simulink model "cps_4_11"  (R2016a)
settings: Solver=VariableStepAuto  StartTime=0.0  StopTime=10.0  RelTol=1e-3
undefined symbols (not defined in the file): sigbuilder_block
libraries: simulink x20
settings Model: Creator=benyett  LastModifiedBy=benyett

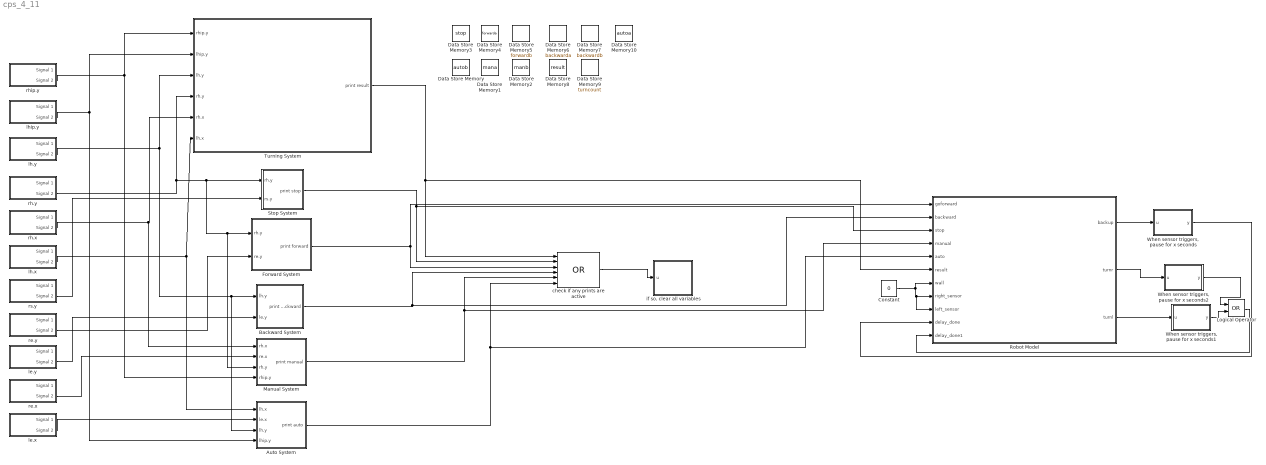
== system cps_4_11 ==
  Auto System : Subsystem
  Backward System : Subsystem
  Constant : Constant  Value=0
  Data Store Memory : DataStoreMemory  DataStoreName=autob  ReadBeforeWriteMsg=warning  WriteAfterWriteMsg=warning  WriteAfterReadMsg=warning  ShowAdditionalParam=off  OutDataTypeStr=double
  Data Store Memory1 : DataStoreMemory  DataStoreName=mana  ReadBeforeWriteMsg=warning  WriteAfterWriteMsg=warning  WriteAfterReadMsg=warning  ShowAdditionalParam=off  OutDataTypeStr=double
  Data Store Memory10 : DataStoreMemory  DataStoreName=autoa  ReadBeforeWriteMsg=warning  WriteAfterWriteMsg=warning  WriteAfterReadMsg=warning  ShowAdditionalParam=off  OutDataTypeStr=double
  Data Store Memory2 : DataStoreMemory  DataStoreName=manb  ReadBeforeWriteMsg=warning  WriteAfterWriteMsg=warning  WriteAfterReadMsg=warning  ShowAdditionalParam=off  OutDataTypeStr=double
  Data Store Memory3 : DataStoreMemory  DataStoreName=stop  ReadBeforeWriteMsg=warning  WriteAfterWriteMsg=warning  WriteAfterReadMsg=warning  ShowAdditionalParam=off  OutDataTypeStr=double
  Data Store Memory4 : DataStoreMemory  DataStoreName=forwarda  ReadBeforeWriteMsg=warning  WriteAfterWriteMsg=warning  WriteAfterReadMsg=warning  ShowAdditionalParam=off  OutDataTypeStr=double
  Data Store Memory5 : DataStoreMemory  DataStoreName=forwardb  ReadBeforeWriteMsg=warning  WriteAfterWriteMsg=warning  WriteAfterReadMsg=warning  ShowAdditionalParam=off  OutDataTypeStr=double
  Data Store Memory6 : DataStoreMemory  DataStoreName=backwarda  ReadBeforeWriteMsg=warning  WriteAfterWriteMsg=warning  WriteAfterReadMsg=warning  ShowAdditionalParam=off  OutDataTypeStr=double
  Data Store Memory7 : DataStoreMemory  DataStoreName=backwardb  ReadBeforeWriteMsg=warning  WriteAfterWriteMsg=warning  WriteAfterReadMsg=warning  ShowAdditionalParam=off  OutDataTypeStr=double
  Data Store Memory8 : DataStoreMemory  DataStoreName=result  ReadBeforeWriteMsg=warning  WriteAfterWriteMsg=warning  WriteAfterReadMsg=warning  ShowAdditionalParam=off  OutDataTypeStr=double
  Data Store Memory9 : DataStoreMemory  DataStoreName=turncount  ReadBeforeWriteMsg=warning  WriteAfterWriteMsg=warning  WriteAfterReadMsg=warning  ShowAdditionalParam=off  OutDataTypeStr=double
  Forward System : Subsystem
  Logical Operator : Logic  Operator=OR  AllPortsSameDT=off  OutDataTypeStr=boolean
  Manual System : Subsystem
  Robot Model : Stateflow chart  TreatAsAtomicUnit=on
  Stop System : Subsystem
  Turning System : Subsystem
  "When sensor triggers, pause for x seconds" : MATLAB Function  TreatAsAtomicUnit=on
  "When sensor triggers, pause for x seconds1" : MATLAB Function  TreatAsAtomicUnit=on
  "When sensor triggers, pause for x seconds2" : MATLAB Function  TreatAsAtomicUnit=on
  check if any prints are active : Logic  Operator=OR  Inputs=6  AllPortsSameDT=off  OutDataTypeStr=boolean
  "if so, clear all variables" : MATLAB Function  TreatAsAtomicUnit=on
  le.x : Subsystem  Tag=STV Subsys  LoadFcn=sigbuilder_block('load');  StartFcn=sigbuilder_block('start');  StopFcn=sigbuilder_block('stop');  ClipboardFcn=sigbuilder_block('clipboard');  mask(Sigbuilder block){}
      mask help: Simulink:masks:SigbuilderBlock_MD
      mask init:
      | if ~strcmp(get_param(bdroot(gcbh),'SimulationStatus'),'stopped') tuvar = sigbuilder_block('maskInit'); end
      settings: CopyFcn=sigbuilder_block('copy');  DeleteFcn=sigbuilder_block('delete');  ModelCloseFcn=sigbuilder_block('modelClose');  PreSaveFcn=sigbuilder_block('preSave');  PauseFcn=sigbuilder_block('pause');  ContinueFcn=sigbuilder_block('continue');  NameChangeFcn=sigbuilder_block('namechange');  OpenFcn=sigbuilder_block('open',[358 196 550 400 ]);  CloseFcn=sigbuilder_block('close');
      mask Display: plot(0, 0, 100, 100,[2, 2, 32, 32, 2], [68, 8, 8, 68, 68],[32, 2], [38, 38], [32, 19, 2],[53, 60, 44], [32, 17, 17, 2],[16, 16, 31, 31]);txt = getActiveGroup(gcbh);text(2, 100, txt,'verticalAlignment', 'top');
  le.y : Subsystem  Tag=STV Subsys  LoadFcn=sigbuilder_block('load');  StartFcn=sigbuilder_block('start');  StopFcn=sigbuilder_block('stop');  ClipboardFcn=sigbuilder_block('clipboard');  mask(Sigbuilder block){}
      mask help: Simulink:masks:SigbuilderBlock_MD
      mask init:
      | if ~strcmp(get_param(bdroot(gcbh),'SimulationStatus'),'stopped') tuvar = sigbuilder_block('maskInit'); end
      settings: CopyFcn=sigbuilder_block('copy');  DeleteFcn=sigbuilder_block('delete');  ModelCloseFcn=sigbuilder_block('modelClose');  PreSaveFcn=sigbuilder_block('preSave');  PauseFcn=sigbuilder_block('pause');  ContinueFcn=sigbuilder_block('continue');  NameChangeFcn=sigbuilder_block('namechange');  OpenFcn=sigbuilder_block('open',[358 196 550 400 ]);  CloseFcn=sigbuilder_block('close');
      mask Display: plot(0, 0, 100, 100,[2, 2, 32, 32, 2], [68, 8, 8, 68, 68],[32, 2], [38, 38], [32, 19, 2],[53, 60, 44], [32, 17, 17, 2],[16, 16, 31, 31]);txt = getActiveGroup(gcbh);text(2, 100, txt,'verticalAlignment', 'top');
  lh.x : Subsystem  Tag=STV Subsys  LoadFcn=sigbuilder_block('load');  StartFcn=sigbuilder_block('start');  StopFcn=sigbuilder_block('stop');  ClipboardFcn=sigbuilder_block('clipboard');  mask(Sigbuilder block){}
      mask help: Simulink:masks:SigbuilderBlock_MD
      mask init:
      | if ~strcmp(get_param(bdroot(gcbh),'SimulationStatus'),'stopped') tuvar = sigbuilder_block('maskInit'); end
      settings: CopyFcn=sigbuilder_block('copy');  DeleteFcn=sigbuilder_block('delete');  ModelCloseFcn=sigbuilder_block('modelClose');  PreSaveFcn=sigbuilder_block('preSave');  PauseFcn=sigbuilder_block('pause');  ContinueFcn=sigbuilder_block('continue');  NameChangeFcn=sigbuilder_block('namechange');  OpenFcn=sigbuilder_block('open',[358 196 550 400 ]);  CloseFcn=sigbuilder_block('close');
      mask Display: plot(0, 0, 100, 100,[2, 2, 32, 32, 2], [68, 8, 8, 68, 68],[32, 2], [38, 38], [32, 19, 2],[53, 60, 44], [32, 17, 17, 2],[16, 16, 31, 31]);txt = getActiveGroup(gcbh);text(2, 100, txt,'verticalAlignment', 'top');
  lh.y : Subsystem  Tag=STV Subsys  LoadFcn=sigbuilder_block('load');  StartFcn=sigbuilder_block('start');  StopFcn=sigbuilder_block('stop');  ClipboardFcn=sigbuilder_block('clipboard');  mask(Sigbuilder block){}
      mask help: Simulink:masks:SigbuilderBlock_MD
      mask init:
      | if ~strcmp(get_param(bdroot(gcbh),'SimulationStatus'),'stopped') tuvar = sigbuilder_block('maskInit'); end
      settings: CopyFcn=sigbuilder_block('copy');  DeleteFcn=sigbuilder_block('delete');  ModelCloseFcn=sigbuilder_block('modelClose');  PreSaveFcn=sigbuilder_block('preSave');  PauseFcn=sigbuilder_block('pause');  ContinueFcn=sigbuilder_block('continue');  NameChangeFcn=sigbuilder_block('namechange');  OpenFcn=sigbuilder_block('open',[358 196 550 400 ]);  CloseFcn=sigbuilder_block('close');
      mask Display: plot(0, 0, 100, 100,[2, 2, 32, 32, 2], [68, 8, 8, 68, 68],[32, 2], [38, 38], [32, 19, 2],[53, 60, 44], [32, 17, 17, 2],[16, 16, 31, 31]);txt = getActiveGroup(gcbh);text(2, 100, txt,'verticalAlignment', 'top');
  lhip.y : Subsystem  Tag=STV Subsys  LoadFcn=sigbuilder_block('load');  StartFcn=sigbuilder_block('start');  StopFcn=sigbuilder_block('stop');  ClipboardFcn=sigbuilder_block('clipboard');  mask(Sigbuilder block){}
      mask help: Simulink:masks:SigbuilderBlock_MD
      mask init:
      | if ~strcmp(get_param(bdroot(gcbh),'SimulationStatus'),'stopped') tuvar = sigbuilder_block('maskInit'); end
      settings: CopyFcn=sigbuilder_block('copy');  DeleteFcn=sigbuilder_block('delete');  ModelCloseFcn=sigbuilder_block('modelClose');  PreSaveFcn=sigbuilder_block('preSave');  PauseFcn=sigbuilder_block('pause');  ContinueFcn=sigbuilder_block('continue');  NameChangeFcn=sigbuilder_block('namechange');  OpenFcn=sigbuilder_block('open',[358 196 550 400 ]);  CloseFcn=sigbuilder_block('close');
      mask Display: plot(0, 0, 100, 100,[2, 2, 32, 32, 2], [68, 8, 8, 68, 68],[32, 2], [38, 38], [32, 19, 2],[53, 60, 44], [32, 17, 17, 2],[16, 16, 31, 31]);txt = getActiveGroup(gcbh);text(2, 100, txt,'verticalAlignment', 'top');
  re.x : Subsystem  Tag=STV Subsys  LoadFcn=sigbuilder_block('load');  StartFcn=sigbuilder_block('start');  StopFcn=sigbuilder_block('stop');  ClipboardFcn=sigbuilder_block('clipboard');  mask(Sigbuilder block){}
      mask help: Simulink:masks:SigbuilderBlock_MD
      mask init:
      | if ~strcmp(get_param(bdroot(gcbh),'SimulationStatus'),'stopped') tuvar = sigbuilder_block('maskInit'); end
      settings: CopyFcn=sigbuilder_block('copy');  DeleteFcn=sigbuilder_block('delete');  ModelCloseFcn=sigbuilder_block('modelClose');  PreSaveFcn=sigbuilder_block('preSave');  PauseFcn=sigbuilder_block('pause');  ContinueFcn=sigbuilder_block('continue');  NameChangeFcn=sigbuilder_block('namechange');  OpenFcn=sigbuilder_block('open',[358 196 550 400 ]);  CloseFcn=sigbuilder_block('close');
      mask Display: plot(0, 0, 100, 100,[2, 2, 32, 32, 2], [68, 8, 8, 68, 68],[32, 2], [38, 38], [32, 19, 2],[53, 60, 44], [32, 17, 17, 2],[16, 16, 31, 31]);txt = getActiveGroup(gcbh);text(2, 100, txt,'verticalAlignment', 'top');
  re.y : Subsystem  Tag=STV Subsys  LoadFcn=sigbuilder_block('load');  StartFcn=sigbuilder_block('start');  StopFcn=sigbuilder_block('stop');  ClipboardFcn=sigbuilder_block('clipboard');  mask(Sigbuilder block){}
      mask help: Simulink:masks:SigbuilderBlock_MD
      mask init:
      | if ~strcmp(get_param(bdroot(gcbh),'SimulationStatus'),'stopped') tuvar = sigbuilder_block('maskInit'); end
      settings: CopyFcn=sigbuilder_block('copy');  DeleteFcn=sigbuilder_block('delete');  ModelCloseFcn=sigbuilder_block('modelClose');  PreSaveFcn=sigbuilder_block('preSave');  PauseFcn=sigbuilder_block('pause');  ContinueFcn=sigbuilder_block('continue');  NameChangeFcn=sigbuilder_block('namechange');  OpenFcn=sigbuilder_block('open',[358 196 550 400 ]);  CloseFcn=sigbuilder_block('close');
      mask Display: plot(0, 0, 100, 100,[2, 2, 32, 32, 2], [68, 8, 8, 68, 68],[32, 2], [38, 38], [32, 19, 2],[53, 60, 44], [32, 17, 17, 2],[16, 16, 31, 31]);txt = getActiveGroup(gcbh);text(2, 100, txt,'verticalAlignment', 'top');
  rh.x : Subsystem  Tag=STV Subsys  LoadFcn=sigbuilder_block('load');  StartFcn=sigbuilder_block('start');  StopFcn=sigbuilder_block('stop');  ClipboardFcn=sigbuilder_block('clipboard');  mask(Sigbuilder block){}
      mask help: Simulink:masks:SigbuilderBlock_MD
      mask init:
      | if ~strcmp(get_param(bdroot(gcbh),'SimulationStatus'),'stopped') tuvar = sigbuilder_block('maskInit'); end
      settings: CopyFcn=sigbuilder_block('copy');  DeleteFcn=sigbuilder_block('delete');  ModelCloseFcn=sigbuilder_block('modelClose');  PreSaveFcn=sigbuilder_block('preSave');  PauseFcn=sigbuilder_block('pause');  ContinueFcn=sigbuilder_block('continue');  NameChangeFcn=sigbuilder_block('namechange');  OpenFcn=sigbuilder_block('open',[358 196 550 400 ]);  CloseFcn=sigbuilder_block('close');
      mask Display: plot(0, 0, 100, 100,[2, 2, 32, 32, 2], [68, 8, 8, 68, 68],[32, 2], [38, 38], [32, 19, 2],[53, 60, 44], [32, 17, 17, 2],[16, 16, 31, 31]);txt = getActiveGroup(gcbh);text(2, 100, txt,'verticalAlignment', 'top');
  rh.y : Subsystem  Tag=STV Subsys  LoadFcn=sigbuilder_block('load');  StartFcn=sigbuilder_block('start');  StopFcn=sigbuilder_block('stop');  ClipboardFcn=sigbuilder_block('clipboard');  mask(Sigbuilder block){}
      mask help: Simulink:masks:SigbuilderBlock_MD
      mask init:
      | if ~strcmp(get_param(bdroot(gcbh),'SimulationStatus'),'stopped') tuvar = sigbuilder_block('maskInit'); end
      settings: CopyFcn=sigbuilder_block('copy');  DeleteFcn=sigbuilder_block('delete');  ModelCloseFcn=sigbuilder_block('modelClose');  PreSaveFcn=sigbuilder_block('preSave');  PauseFcn=sigbuilder_block('pause');  ContinueFcn=sigbuilder_block('continue');  NameChangeFcn=sigbuilder_block('namechange');  OpenFcn=sigbuilder_block('open',[358 196 550 400 ]);  CloseFcn=sigbuilder_block('close');
      mask Display: plot(0, 0, 100, 100,[2, 2, 32, 32, 2], [68, 8, 8, 68, 68],[32, 2], [38, 38], [32, 19, 2],[53, 60, 44], [32, 17, 17, 2],[16, 16, 31, 31]);txt = getActiveGroup(gcbh);text(2, 100, txt,'verticalAlignment', 'top');
  rhip.y : Subsystem  Tag=STV Subsys  LoadFcn=sigbuilder_block('load');  StartFcn=sigbuilder_block('start');  StopFcn=sigbuilder_block('stop');  ClipboardFcn=sigbuilder_block('clipboard');  mask(Sigbuilder block){}
      mask help: Simulink:masks:SigbuilderBlock_MD
      mask init:
      | if ~strcmp(get_param(bdroot(gcbh),'SimulationStatus'),'stopped') tuvar = sigbuilder_block('maskInit'); end
      settings: CopyFcn=sigbuilder_block('copy');  DeleteFcn=sigbuilder_block('delete');  ModelCloseFcn=sigbuilder_block('modelClose');  PreSaveFcn=sigbuilder_block('preSave');  PauseFcn=sigbuilder_block('pause');  ContinueFcn=sigbuilder_block('continue');  NameChangeFcn=sigbuilder_block('namechange');  OpenFcn=sigbuilder_block('open',[358 196 550 400 ]);  CloseFcn=sigbuilder_block('close');
      mask Display: plot(0, 0, 100, 100,[2, 2, 32, 32, 2], [68, 8, 8, 68, 68],[32, 2], [38, 38], [32, 19, 2],[53, 60, 44], [32, 17, 17, 2],[16, 16, 31, 31]);txt = getActiveGroup(gcbh);text(2, 100, txt,'verticalAlignment', 'top');
  rs.y : Subsystem  Tag=STV Subsys  LoadFcn=sigbuilder_block('load');  StartFcn=sigbuilder_block('start');  StopFcn=sigbuilder_block('stop');  ClipboardFcn=sigbuilder_block('clipboard');  mask(Sigbuilder block){}
      mask help: Simulink:masks:SigbuilderBlock_MD
      mask init:
      | if ~strcmp(get_param(bdroot(gcbh),'SimulationStatus'),'stopped') tuvar = sigbuilder_block('maskInit'); end
      settings: CopyFcn=sigbuilder_block('copy');  DeleteFcn=sigbuilder_block('delete');  ModelCloseFcn=sigbuilder_block('modelClose');  PreSaveFcn=sigbuilder_block('preSave');  PauseFcn=sigbuilder_block('pause');  ContinueFcn=sigbuilder_block('continue');  NameChangeFcn=sigbuilder_block('namechange');  OpenFcn=sigbuilder_block('open',[358 196 550 400 ]);  CloseFcn=sigbuilder_block('close');
      mask Display: plot(0, 0, 100, 100,[2, 2, 32, 32, 2], [68, 8, 8, 68, 68],[32, 2], [38, 38], [32, 19, 2],[53, 60, 44], [32, 17, 17, 2],[16, 16, 31, 31]);txt = getActiveGroup(gcbh);text(2, 100, txt,'verticalAlignment', 'top');
  wires:
  Turning System/1(print result) -> Robot Model/6(result), check if any prints are active/1
  Stop System/1(print stop) -> Robot Model/3(stop), check if any prints are active/2
  Forward System/1(print forward) -> Robot Model/1(goforward), check if any prints are active/3
  Backward System/1(print backward) -> Robot Model/2(backward), check if any prints are active/4
  Manual System/1(print manual) -> Robot Model/4(manual), check if any prints are active/5
  Auto System/1(print auto) -> Robot Model/5(auto), check if any prints are active/6
  check if any prints are active/1 -> "if so, clear all variables"/1(u)
  rhip.y/2(Signal 2) -> Manual System/4(rhip.y), Turning System/1(rhip.y)
  lhip.y/2(Signal 2) -> Auto System/4(lhip.y), Turning System/2(lhip.y)
  lh.y/2(Signal 2) -> Auto System/3(lh.y), Backward System/1(lh.y), Turning System/3(lh.y)
  rh.y/2(Signal 2) -> Manual System/3(rh.y), Forward System/1(rh.y), Stop System/1(rh.y), Turning System/4(rh.y)
  rh.x/2(Signal 2) -> Manual System/1(rh.x), Turning System/5(rh.x)
  lh.x/2(Signal 2) -> Auto System/1(lh.x), Turning System/6(lh.x)
  rs.y/2(Signal 2) -> Stop System/2(rs.y)
  re.y/2(Signal 2) -> Forward System/2(re.y)
  le.y/2(Signal 2) -> Backward System/2(le.y)
  re.x/2(Signal 2) -> Manual System/2(re.x)
  le.x/2(Signal 2) -> Auto System/2(le.x)
  "When sensor triggers, pause for x seconds"/1(y) -> Robot Model/10(delay_done)
  Robot Model/1(backup) -> "When sensor triggers, pause for x seconds"/1(u)
  Robot Model/2(turnr) -> "When sensor triggers, pause for x seconds2"/1(u)
  Robot Model/3(turnl) -> "When sensor triggers, pause for x seconds1"/1(u)
  Constant/1 -> Robot Model/9(left_sensor), Robot Model/8(right_sensor), Robot Model/7(wall)
  "When sensor triggers, pause for x seconds2"/1(y) -> Logical Operator/1
  "When sensor triggers, pause for x seconds1"/1(y) -> Logical Operator/2
  Logical Operator/1 -> Robot Model/11(delay_done1)

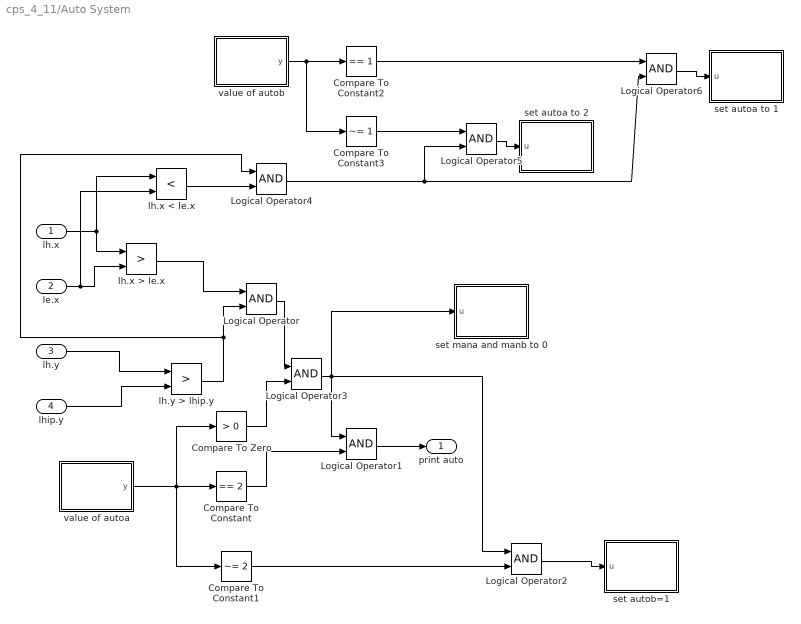
== system cps_4_11/Auto System ==
  lh.x : Inport
  le.x : Inport  Port=2
  lh.y : Inport  Port=3
  lhip.y : Inport  Port=4
  Compare To Constant : simulink/Logic and Bit Operations/Compare To Constant  relop===  const=2  OutDataTypeStr=boolean
  Compare To Constant1 : simulink/Logic and Bit Operations/Compare To Constant  relop=~=  const=2  OutDataTypeStr=boolean
  Compare To Constant2 : simulink/Logic and Bit Operations/Compare To Constant  relop===  const=1  OutDataTypeStr=boolean
  Compare To Constant3 : simulink/Logic and Bit Operations/Compare To Constant  relop=~=  const=1  OutDataTypeStr=boolean
  Compare To Zero : simulink/Logic and Bit Operations/Compare To Zero  relop=>  OutDataTypeStr=boolean
  Logical Operator{,1..6} (7 alike) : Logic  AllPortsSameDT=off  OutDataTypeStr=boolean
  lh.x < le.x : RelationalOperator  Operator=<  OutDataTypeStr=boolean
  lh.x > le.x : RelationalOperator  Operator=>  OutDataTypeStr=boolean
  lh.y > lhip.y : RelationalOperator  Operator=>  OutDataTypeStr=boolean
  set autoa to 1 : MATLAB Function  TreatAsAtomicUnit=on
  set autoa to 2 : MATLAB Function  TreatAsAtomicUnit=on
  set autob=1 : MATLAB Function  TreatAsAtomicUnit=on
  set mana and manb to 0 : MATLAB Function  TreatAsAtomicUnit=on
  value of autoa : MATLAB Function  TreatAsAtomicUnit=on
  value of autob : MATLAB Function  TreatAsAtomicUnit=on
  print auto : Outport
  wires:
  le.x/1 -> lh.x < le.x/2, lh.x > le.x/2
  lh.x/1 -> lh.x < le.x/1, lh.x > le.x/1
  lhip.y/1 -> lh.y > lhip.y/2
  lh.y/1 -> lh.y > lhip.y/1
  lh.x > le.x/1 -> Logical Operator/1
  lh.y > lhip.y/1 -> Logical Operator4/1, Logical Operator/2
  Logical Operator/1 -> Logical Operator3/1
  value of autoa/1(y) -> Compare To Zero/1, Compare To Constant1/1, Compare To Constant/1
  Compare To Constant/1 -> Logical Operator1/2
  Compare To Constant1/1 -> Logical Operator2/2
  Logical Operator1/1 -> print auto/1
  Logical Operator2/1 -> set autob=1/1(u)
  Logical Operator3/1 -> set mana and manb to 0/1(u), Logical Operator1/1, Logical Operator2/1
  Compare To Zero/1 -> Logical Operator3/2
  lh.x < le.x/1 -> Logical Operator4/2
  value of autob/1(y) -> Compare To Constant3/1, Compare To Constant2/1
  Compare To Constant3/1 -> Logical Operator5/1
  Compare To Constant2/1 -> Logical Operator6/1
  Logical Operator4/1 -> Logical Operator5/2, Logical Operator6/2
  Logical Operator5/1 -> set autoa to 2/1(u)
  Logical Operator6/1 -> set autoa to 1/1(u)

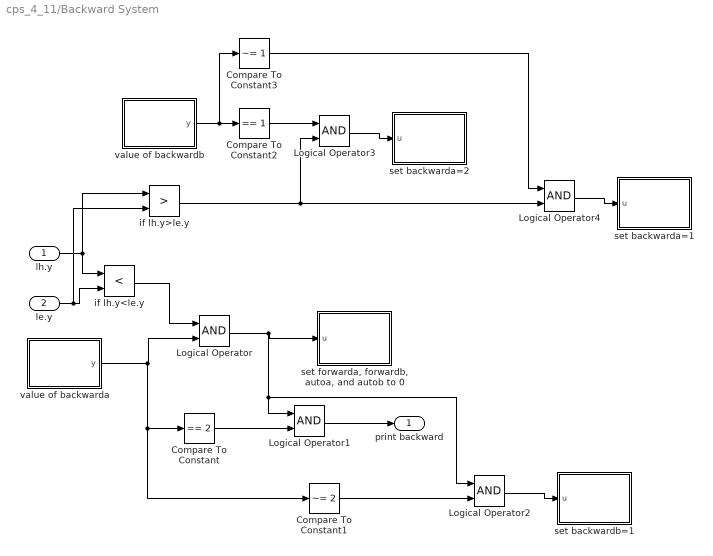
== system cps_4_11/Backward System ==
  lh.y : Inport
  le.y : Inport  Port=2
  Compare To Constant : simulink/Logic and Bit Operations/Compare To Constant  relop===  const=2  OutDataTypeStr=boolean
  Compare To Constant1 : simulink/Logic and Bit Operations/Compare To Constant  relop=~=  const=2  OutDataTypeStr=boolean
  Compare To Constant2 : simulink/Logic and Bit Operations/Compare To Constant  relop===  const=1  OutDataTypeStr=boolean
  Compare To Constant3 : simulink/Logic and Bit Operations/Compare To Constant  relop=~=  const=1  OutDataTypeStr=boolean
  Logical Operator{,1..4} (5 alike) : Logic  AllPortsSameDT=off  OutDataTypeStr=boolean
  if lh.y<le.y : RelationalOperator  Operator=<  OutDataTypeStr=boolean
  if lh.y>le.y : RelationalOperator  Operator=>  OutDataTypeStr=boolean
  set backwarda=1 : MATLAB Function  TreatAsAtomicUnit=on
  set backwarda=2 : MATLAB Function  TreatAsAtomicUnit=on
  set backwardb=1 : MATLAB Function  TreatAsAtomicUnit=on
  "set forwarda, forwardb, autoa, and autob to 0" : MATLAB Function  TreatAsAtomicUnit=on
  value of backwarda : MATLAB Function  TreatAsAtomicUnit=on
  value of backwardb : MATLAB Function  TreatAsAtomicUnit=on
  print backward : Outport
  wires:
  le.y/1 -> if lh.y>le.y/2, if lh.y<le.y/2
  lh.y/1 -> if lh.y>le.y/1, if lh.y<le.y/1
  if lh.y<le.y/1 -> Logical Operator/1
  value of backwarda/1(y) -> Compare To Constant1/1, Compare To Constant/1, Logical Operator/2
  Logical Operator/1 -> Logical Operator2/1, Logical Operator1/1, "set forwarda, forwardb, autoa, and autob to 0"/1(u)
  Compare To Constant/1 -> Logical Operator1/2
  Logical Operator1/1 -> print backward/1
  Compare To Constant1/1 -> Logical Operator2/2
  Logical Operator2/1 -> set backwardb=1/1(u)
  value of backwardb/1(y) -> Compare To Constant3/1, Compare To Constant2/1
  if lh.y>le.y/1 -> Logical Operator3/2, Logical Operator4/2
  Compare To Constant2/1 -> Logical Operator3/1
  Compare To Constant3/1 -> Logical Operator4/1
  Logical Operator4/1 -> set backwarda=1/1(u)
  Logical Operator3/1 -> set backwarda=2/1(u)

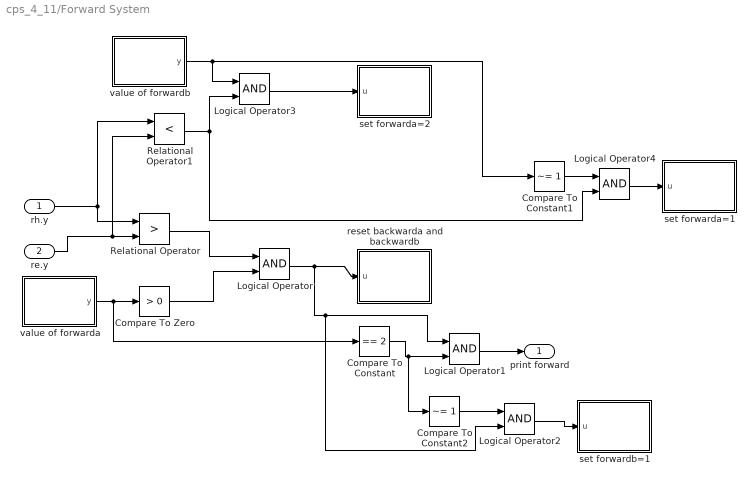
== system cps_4_11/Forward System ==
  rh.y : Inport
  re.y : Inport  Port=2
  Compare To Constant : simulink/Logic and Bit Operations/Compare To Constant  relop===  const=2  OutDataTypeStr=boolean
  Compare To Constant1 : simulink/Logic and Bit Operations/Compare To Constant  relop=~=  const=1  OutDataTypeStr=boolean
  Compare To Constant2 : simulink/Logic and Bit Operations/Compare To Constant  relop=~=  const=1  OutDataTypeStr=boolean
  Compare To Zero : simulink/Logic and Bit Operations/Compare To Zero  relop=>  OutDataTypeStr=boolean
  Logical Operator{,1..4} (5 alike) : Logic  AllPortsSameDT=off  OutDataTypeStr=boolean
  Relational Operator : RelationalOperator  Operator=>  OutDataTypeStr=boolean
  Relational Operator1 : RelationalOperator  Operator=<  OutDataTypeStr=boolean
  reset backwarda and backwardb : MATLAB Function  TreatAsAtomicUnit=on
  set forwarda=1 : MATLAB Function  TreatAsAtomicUnit=on
  set forwarda=2 : MATLAB Function  TreatAsAtomicUnit=on
  set forwardb=1 : MATLAB Function  TreatAsAtomicUnit=on
  value of forwarda : MATLAB Function  TreatAsAtomicUnit=on
  value of forwardb : MATLAB Function  TreatAsAtomicUnit=on
  print forward : Outport
  wires:
  Compare To Zero/1 -> Logical Operator/2
  value of forwarda/1(y) -> Compare To Constant/1, Compare To Zero/1
  re.y/1 -> Relational Operator1/2, Relational Operator/2
  rh.y/1 -> Relational Operator1/1, Relational Operator/1
  Relational Operator/1 -> Logical Operator/1
  Logical Operator/1 -> Logical Operator2/2, Logical Operator1/1, reset backwarda and backwardb/1(u)
  Compare To Constant/1 -> Compare To Constant2/1, Logical Operator1/2
  Logical Operator1/1 -> print forward/1
  Compare To Constant2/1 -> Logical Operator2/1
  Logical Operator2/1 -> set forwardb=1/1(u)
  value of forwardb/1(y) -> Compare To Constant1/1, Logical Operator3/1
  Relational Operator1/1 -> Logical Operator4/2, Logical Operator3/2
  Logical Operator3/1 -> set forwarda=2/1(u)
  Compare To Constant1/1 -> Logical Operator4/1
  Logical Operator4/1 -> set forwarda=1/1(u)

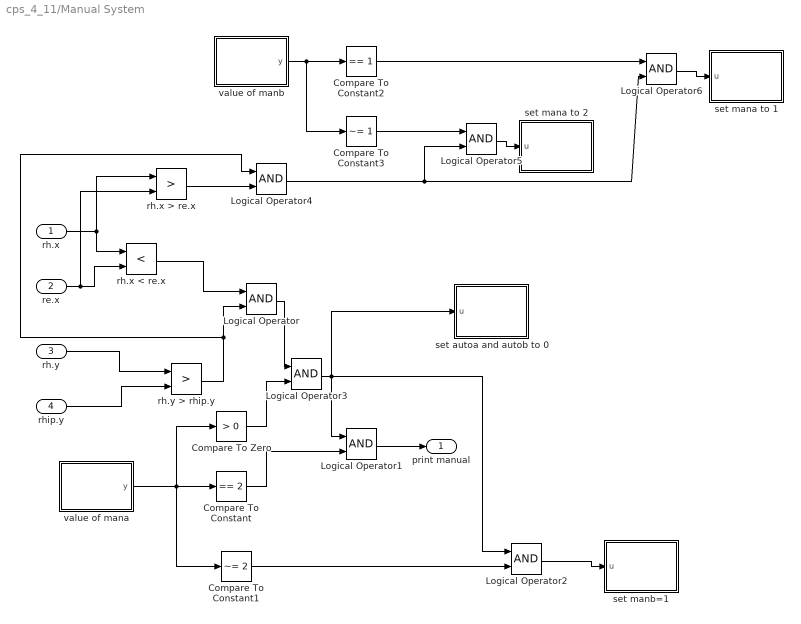
== system cps_4_11/Manual System ==
  rh.x : Inport
  re.x : Inport  Port=2
  rh.y : Inport  Port=3
  rhip.y : Inport  Port=4
  Compare To Constant : simulink/Logic and Bit Operations/Compare To Constant  relop===  const=2  OutDataTypeStr=boolean
  Compare To Constant1 : simulink/Logic and Bit Operations/Compare To Constant  relop=~=  const=2  OutDataTypeStr=boolean
  Compare To Constant2 : simulink/Logic and Bit Operations/Compare To Constant  relop===  const=1  OutDataTypeStr=boolean
  Compare To Constant3 : simulink/Logic and Bit Operations/Compare To Constant  relop=~=  const=1  OutDataTypeStr=boolean
  Compare To Zero : simulink/Logic and Bit Operations/Compare To Zero  relop=>  OutDataTypeStr=boolean
  Logical Operator{,1..6} (7 alike) : Logic  AllPortsSameDT=off  OutDataTypeStr=boolean
  rh.x < re.x : RelationalOperator  Operator=<  OutDataTypeStr=boolean
  rh.x > re.x : RelationalOperator  Operator=>  OutDataTypeStr=boolean
  rh.y > rhip.y : RelationalOperator  Operator=>  OutDataTypeStr=boolean
  set autoa and autob to 0 : MATLAB Function  TreatAsAtomicUnit=on
  set mana to 1 : MATLAB Function  TreatAsAtomicUnit=on
  set mana to 2 : MATLAB Function  TreatAsAtomicUnit=on
  set manb=1 : MATLAB Function  TreatAsAtomicUnit=on
  value of mana : MATLAB Function  TreatAsAtomicUnit=on
  value of manb : MATLAB Function  TreatAsAtomicUnit=on
  print manual : Outport
  wires:
  Logical Operator6/1 -> set mana to 1/1(u)
  Logical Operator5/1 -> set mana to 2/1(u)
  Logical Operator4/1 -> Logical Operator6/2, Logical Operator5/2
  Compare To Constant2/1 -> Logical Operator6/1
  Compare To Constant3/1 -> Logical Operator5/1
  value of manb/1(y) -> Compare To Constant2/1, Compare To Constant3/1
  rh.x > re.x/1 -> Logical Operator4/2
  Compare To Zero/1 -> Logical Operator3/2
  Logical Operator3/1 -> Logical Operator2/1, Logical Operator1/1, set autoa and autob to 0/1(u)
  Logical Operator2/1 -> set manb=1/1(u)
  Logical Operator1/1 -> print manual/1
  Compare To Constant1/1 -> Logical Operator2/2
  Compare To Constant/1 -> Logical Operator1/2
  value of mana/1(y) -> Compare To Constant/1, Compare To Constant1/1, Compare To Zero/1
  Logical Operator/1 -> Logical Operator3/1
  rh.y > rhip.y/1 -> Logical Operator/2, Logical Operator4/1
  rh.x < re.x/1 -> Logical Operator/1
  rh.y/1 -> rh.y > rhip.y/1
  rhip.y/1 -> rh.y > rhip.y/2
  rh.x/1 -> rh.x < re.x/1, rh.x > re.x/1
  re.x/1 -> rh.x < re.x/2, rh.x > re.x/2

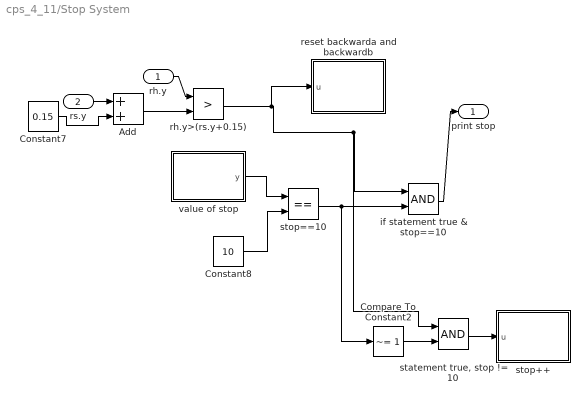
== system cps_4_11/Stop System ==
  rh.y : Inport
  rs.y : Inport  Port=2
  Add : Sum
  Compare To Constant2 : simulink/Logic and Bit Operations/Compare To Constant  relop=~=  const=1  OutDataTypeStr=boolean
  Constant7 : Constant  Value=0.15
  Constant8 : Constant  Value=10
  if statement true & stop==10 : Logic  AllPortsSameDT=off  OutDataTypeStr=boolean
  reset backwarda and backwardb : MATLAB Function  TreatAsAtomicUnit=on
  rh.y>(rs.y+0.15) : RelationalOperator  Operator=>  OutDataTypeStr=boolean
  "statement true, stop != 10" : Logic  AllPortsSameDT=off  OutDataTypeStr=boolean
  stop++ : MATLAB Function  TreatAsAtomicUnit=on
  stop==10 : RelationalOperator  Operator===  OutDataTypeStr=boolean
  value of stop : MATLAB Function  TreatAsAtomicUnit=on
  print stop : Outport
  wires:
  stop==10/1 -> Compare To Constant2/1, if statement true & stop==10/2
  rs.y/1 -> Add/1
  Add/1 -> rh.y>(rs.y+0.15)/2
  Constant7/1 -> Add/2
  rh.y/1 -> rh.y>(rs.y+0.15)/1
  value of stop/1(y) -> stop==10/1
  Constant8/1 -> stop==10/2
  rh.y>(rs.y+0.15)/1 -> reset backwarda and backwardb/1(u), "statement true, stop != 10"/1, if statement true & stop==10/1
  if statement true & stop==10/1 -> print stop/1
  Compare To Constant2/1 -> "statement true, stop != 10"/2
  "statement true, stop != 10"/1 -> stop++/1(u)

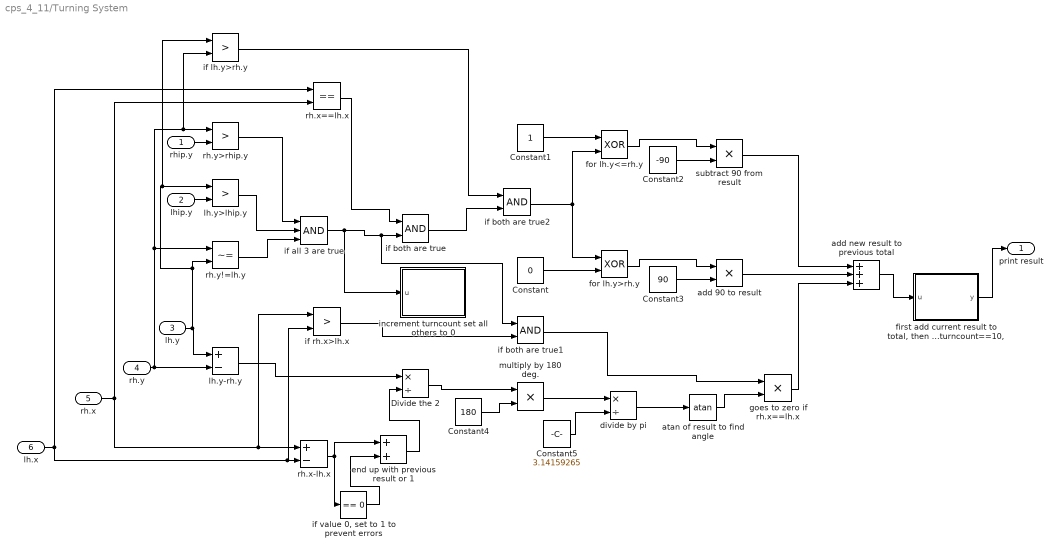
== system cps_4_11/Turning System ==
  rhip.y : Inport
  lhip.y : Inport  Port=2
  lh.y : Inport  Port=3
  rh.y : Inport  Port=4
  rh.x : Inport  Port=5
  lh.x : Inport  Port=6
  Constant : Constant  Value=0
  Constant1 : Constant
  Constant2 : Constant  Value=-90
  Constant3 : Constant  Value=90
  Constant4 : Constant  Value=180
  Constant5 : Constant  Value=3.14159265
  Divide the 2 : Product  Inputs=*/
  add 90 to result : Product
  add new result to previous total : Sum  Inputs=+++
  atan of result to find angle : Trigonometry  Operator=atan
  divide by pi : Product  Inputs=*/
  end up with previous result or 1 : Sum
  "first add current result to total, then if turncount==10, " : MATLAB Function  TreatAsAtomicUnit=on
  for lh.y<=rh.y : Logic  Operator=XOR  AllPortsSameDT=off  OutDataTypeStr=boolean
  for lh.y>rh.y : Logic  Operator=XOR  AllPortsSameDT=off  OutDataTypeStr=boolean
  goes to zero if rh.x==lh.x : Product
  if all 3 are true : Logic  Inputs=3  AllPortsSameDT=off  OutDataTypeStr=boolean
  if both are true : Logic  AllPortsSameDT=off  OutDataTypeStr=boolean
  if both are true1 : Logic  AllPortsSameDT=off  OutDataTypeStr=boolean
  if both are true2 : Logic  AllPortsSameDT=off  OutDataTypeStr=boolean
  if lh.y>rh.y : RelationalOperator  Operator=>  OutDataTypeStr=boolean
  if rh.x>lh.x : RelationalOperator  Operator=>  OutDataTypeStr=boolean
  "if value 0, set to 1 to prevent errors" : simulink/Logic and Bit Operations/Compare To Zero  relop===  OutDataTypeStr=boolean
  increment turncount set all others to 0 : MATLAB Function  TreatAsAtomicUnit=on
  lh.y-rh.y : Sum  Inputs=+-
  lh.y>lhip.y : RelationalOperator  Operator=>  OutDataTypeStr=boolean
  multiply by 180 deg. : Product
  rh.x-lh.x : Sum  Inputs=+-
  rh.x==lh.x : RelationalOperator  Operator===  OutDataTypeStr=boolean
  rh.y!=lh.y : RelationalOperator  Operator=~=  OutDataTypeStr=boolean
  rh.y>rhip.y : RelationalOperator  Operator=>  OutDataTypeStr=boolean
  subtract 90 from result : Product
  print result : Outport
  wires:
  rhip.y/1 -> rh.y>rhip.y/2
  rh.x/1 -> rh.x==lh.x/2, if rh.x>lh.x/1, rh.x-lh.x/1
  lh.x/1 -> rh.x==lh.x/1, if rh.x>lh.x/2, rh.x-lh.x/2
  "first add current result to total, then if turncount==10, "/1(y) -> print result/1
  lhip.y/1 -> lh.y>lhip.y/2
  lh.y/1 -> rh.y!=lh.y/2, if lh.y>rh.y/1, lh.y>lhip.y/1, lh.y-rh.y/1
  rh.y/1 -> if lh.y>rh.y/2, rh.y>rhip.y/1, rh.y!=lh.y/1, lh.y-rh.y/2
  rh.y>rhip.y/1 -> if all 3 are true/1
  lh.y>lhip.y/1 -> if all 3 are true/2
  rh.y!=lh.y/1 -> if all 3 are true/3
  rh.x==lh.x/1 -> if both are true/1
  if all 3 are true/1 -> increment turncount set all others to 0/1(u), if both are true1/1, if both are true/2
  if both are true/1 -> if both are true2/2
  if lh.y>rh.y/1 -> if both are true2/1
  Constant1/1 -> for lh.y<=rh.y/1
  if both are true2/1 -> for lh.y>rh.y/1, for lh.y<=rh.y/2
  Constant/1 -> for lh.y>rh.y/2
  for lh.y>rh.y/1 -> add 90 to result/1
  Constant3/1 -> add 90 to result/2
  for lh.y<=rh.y/1 -> subtract 90 from result/1
  Constant2/1 -> subtract 90 from result/2
  if rh.x>lh.x/1 -> if both are true1/2
  lh.y-rh.y/1 -> Divide the 2/1
  Constant4/1 -> multiply by 180 deg./2
  Divide the 2/1 -> multiply by 180 deg./1
  Constant5/1 -> divide by pi/2
  multiply by 180 deg./1 -> divide by pi/1
  divide by pi/1 -> atan of result to find angle/1
  if both are true1/1 -> goes to zero if rh.x==lh.x/1
  atan of result to find angle/1 -> goes to zero if rh.x==lh.x/2
  subtract 90 from result/1 -> add new result to previous total/1
  add 90 to result/1 -> add new result to previous total/2
  goes to zero if rh.x==lh.x/1 -> add new result to previous total/3
  add new result to previous total/1 -> "first add current result to total, then if turncount==10, "/1(u)
  rh.x-lh.x/1 -> "if value 0, set to 1 to prevent errors"/1, end up with previous result or 1/1
  end up with previous result or 1/1 -> Divide the 2/2
  "if value 0, set to 1 to prevent errors"/1 -> end up with previous result or 1/2

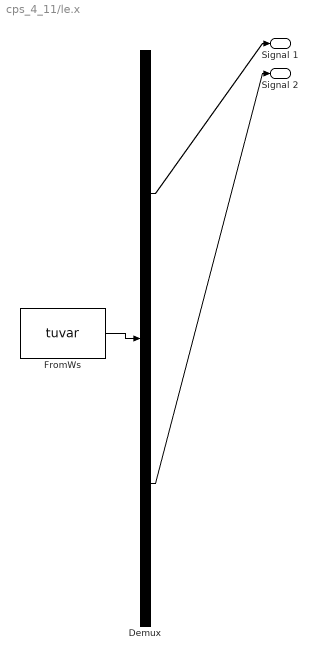
== system cps_4_11/le.x ==
  Demux : Demux  Tag=STV Demux  Outputs=2
  FromWs : FromWorkspace  Tag=STV FromWs  VariableName=tuvar  SampleTime=0
      SigBuilderData=|
      | common.afterFinalStr = 'Extrapolate'
      | common.sampleTime = 0
      | dataSet.timeRange = [0 10]
      | dataSet.name = 'Group 1'
      | sbobj.Groups.Name = 'Group 1'
      | sbobj.Groups.Signals(1).Name = 'Signal 1'
      | sbobj.Groups.Signals(1).XData = [0 0.11 0.2 0.33 0.45 0.62 0.62 0.81 0.81 1 1.12 1.29 1.41 1.61 1.76 1.85 1.96 2.05 2.19 2.19 2.33 2.33 2.45 2.45 2.6 2.6 2.73 2.92 3.05 3.24 3.24 3.41 3.41 3.6 3.6 3.81 4 4.1 4.1 4.23 4.23 4.4 4.55 4.55 4.73 4.73 4.89 5.01 5.17 5.39 5.54 5.75 5.89 6 6 6.15 6.15 6.28 6.28 6.45 6.45 6.63 6.63 6.83 6.83 7.05 7.15 7.15 7.31 7.31 7.42 7.59 7.76 7.95 8.13 8.26 8.26 8.42 8.42 8.62 8.78 8.96 9.1 9.31 9.48 9.72 9.89 10]
      | sbobj.Groups.Signals(1).YData = [0 0 0.205 0 0 0 0.1595 0.1595 0 0 0 -0.033 0 0 0.273 0 0 0 0 0.3025 0.3025 0 0 0.32 0.32 0 0 0.197 0 0 0.045 0.045 -0.09 -0.09 0 0 0 0 -0.204 -0.204 0 0 0 0.238 0.238 0 0 -0.2 0 0 0.374 0 0 0 -0.034 -0.034 0 0 0.275 0.275 0 0 -0.265 -0.265 0 0.096 0 -0.166 -0.166 0 0 0.254 0 0 0 0 0.403 0.403 0 0 0 0 -0.054 0 0 0.172 0 0]
      | sbobj.Groups.Signals(2).Name = 'Signal 2'
      | sbobj.Groups.Signals(2).XData = [0 10]
      | sbobj.Groups.Signals(2).YData = [0 0]
  Signal 1 : Outport  Tag=STV Outport
  Signal 2 : Outport  Tag=STV Outport  Port=2
  wires:
  FromWs/1 -> Demux/1
  Demux/1 -> Signal 1/1
  Demux/2 -> Signal 2/1

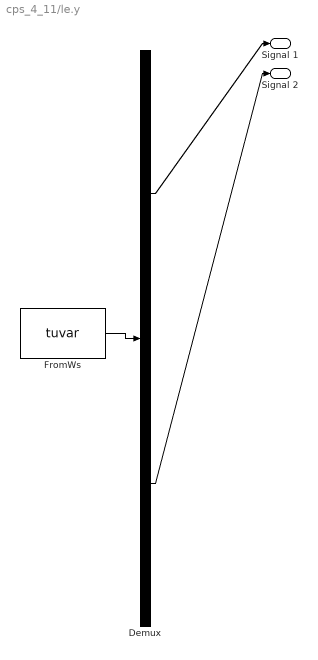
== system cps_4_11/le.y ==
  Demux : Demux  Tag=STV Demux  Outputs=2
  FromWs : FromWorkspace  Tag=STV FromWs  VariableName=tuvar  SampleTime=0
      SigBuilderData=|
      | common.afterFinalStr = 'Extrapolate'
      | common.sampleTime = 0
      | dataSet.timeRange = [0 10]
      | dataSet.name = 'Group 1'
      | sbobj.Groups.Name = 'Group 1'
      | sbobj.Groups.Signals(1).Name = 'Signal 1'
      | sbobj.Groups.Signals(1).XData = [0 0.11 0.2 0.33 0.45 0.62 0.62 0.81 0.81 1 1.12 1.29 1.41 1.61 1.76 1.85 1.96 2.05 2.19 2.19 2.33 2.33 2.45 2.45 2.6 2.6 2.73 2.92 3.05 3.24 3.24 3.41 3.41 3.6 3.6 3.81 4 4.1 4.1 4.23 4.23 4.4 4.55 4.55 4.73 4.73 4.89 5.01 5.17 5.39 5.54 5.75 5.89 6 6 6.15 6.15 6.28 6.28 6.45 6.45 6.63 6.63 6.83 6.83 7.05 7.15 7.15 7.31 7.31 7.42 7.59 7.76 7.95 8.13 8.26 8.26 8.42 8.42 8.62 8.78 8.96 9.1 9.31 9.48 9.72 9.89 10]
      | sbobj.Groups.Signals(1).YData = [0 0 0.205 0 0 0 0.1595 0.1595 0 0 0 -0.033 0 0 0.273 0 0 0 0 0.3025 0.3025 0 0 0.32 0.32 0 0 0.197 0 0 0.045 0.045 -0.09 -0.09 0 0 0 0 -0.204 -0.204 0 0 0 0.238 0.238 0 0 -0.2 0 0 0.374 0 0 0 -0.034 -0.034 0 0 0.275 0.275 0 0 -0.265 -0.265 0 0.096 0 -0.166 -0.166 0 0 0.254 0 0 0 0 0.403 0.403 0 0 0 0 -0.054 0 0 0.172 0 0]
      | sbobj.Groups.Signals(2).Name = 'Signal 2'
      | sbobj.Groups.Signals(2).XData = [0 10]
      | sbobj.Groups.Signals(2).YData = [0 0]
  Signal 1 : Outport  Tag=STV Outport
  Signal 2 : Outport  Tag=STV Outport  Port=2
  wires:
  FromWs/1 -> Demux/1
  Demux/1 -> Signal 1/1
  Demux/2 -> Signal 2/1

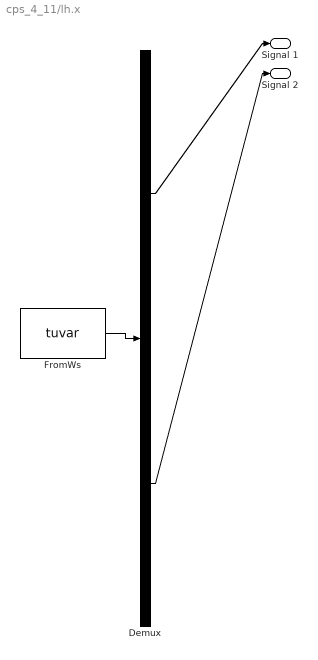
== system cps_4_11/lh.x ==
  Demux : Demux  Tag=STV Demux  Outputs=2
  FromWs : FromWorkspace  Tag=STV FromWs  VariableName=tuvar  SampleTime=0
      SigBuilderData=|
      | common.afterFinalStr = 'Extrapolate'
      | common.sampleTime = 0
      | dataSet.timeRange = [0 10]
      | dataSet.name = 'Group 1'
      | sbobj.Groups.Name = 'Group 1'
      | sbobj.Groups.Signals(1).Name = 'Signal 1'
      | sbobj.Groups.Signals(1).XData = [0 0.11 0.2 0.33 0.45 0.62 0.62 0.81 0.81 1 1.12 1.29 1.41 1.61 1.76 1.85 1.96 2.05 2.19 2.19 2.33 2.33 2.45 2.45 2.6 2.6 2.73 2.92 3.05 3.24 3.24 3.41 3.41 3.6 3.6 3.81 4 4.1 4.1 4.23 4.23 4.4 4.55 4.55 4.73 4.73 4.89 5.01 5.17 5.39 5.54 5.75 5.89 6 6 6.15 6.15 6.28 6.28 6.45 6.45 6.63 6.63 6.83 6.83 7.05 7.15 7.15 7.31 7.31 7.42 7.59 7.76 7.95 8.13 8.26 8.26 8.42 8.42 8.62 8.78 8.96 9.1 9.31 9.48 9.72 9.89 10]
      | sbobj.Groups.Signals(1).YData = [0 0 0.205 0 0 0 0.1595 0.1595 0 0 0 -0.033 0 0 0.273 0 0 0 0 0.3025 0.3025 0 0 0.32 0.32 0 0 0.197 0 0 0.045 0.045 -0.09 -0.09 0 0 0 0 -0.204 -0.204 0 0 0 0.238 0.238 0 0 -0.2 0 0 0.374 0 0 0 -0.034 -0.034 0 0 0.275 0.275 0 0 -0.265 -0.265 0 0.096 0 -0.166 -0.166 0 0 0.254 0 0 0 0 0.403 0.403 0 0 0 0 -0.054 0 0 0.172 0 0]
      | sbobj.Groups.Signals(2).Name = 'Signal 2'
      | sbobj.Groups.Signals(2).XData = [0 10]
      | sbobj.Groups.Signals(2).YData = [0 0]
  Signal 1 : Outport  Tag=STV Outport
  Signal 2 : Outport  Tag=STV Outport  Port=2
  wires:
  Demux/1 -> Signal 1/1
  FromWs/1 -> Demux/1
  Demux/2 -> Signal 2/1

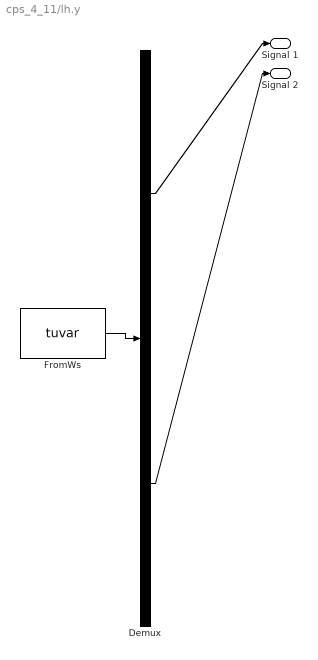
== system cps_4_11/lh.y ==
  Demux : Demux  Tag=STV Demux  Outputs=2
  FromWs : FromWorkspace  Tag=STV FromWs  VariableName=tuvar  SampleTime=0
      SigBuilderData=|
      | common.afterFinalStr = 'Extrapolate'
      | common.sampleTime = 0
      | dataSet.timeRange = [0 10]
      | dataSet.name = 'Group 1'
      | sbobj.Groups.Name = 'Group 1'
      | sbobj.Groups.Signals(1).Name = 'Signal 1'
      | sbobj.Groups.Signals(1).XData = [0 0.11 0.2 0.33 0.45 0.62 0.62 0.81 0.81 1 1.12 1.29 1.41 1.61 1.76 1.85 1.96 2.05 2.19 2.19 2.33 2.33 2.45 2.45 2.6 2.6 2.73 2.92 3.05 3.24 3.24 3.41 3.41 3.6 3.6 3.81 4 4.1 4.1 4.23 4.23 4.4 4.55 4.55 4.73 4.73 4.89 5.01 5.17 5.39 5.54 5.75 5.89 6 6 6.15 6.15 6.28 6.28 6.45 6.45 6.63 6.63 6.83 6.83 7.05 7.15 7.15 7.31 7.31 7.42 7.59 7.76 7.95 8.13 8.26 8.26 8.42 8.42 8.62 8.78 8.96 9.1 9.31 9.48 9.72 9.89 10]
      | sbobj.Groups.Signals(1).YData = [0 0 0.205 0 0 0 0.1595 0.1595 0 0 0 -0.033 0 0 0.273 0 0 0 0 0.3025 0.3025 0 0 0.32 0.32 0 0 0.197 0 0 0.045 0.045 -0.09 -0.09 0 0 0 0 -0.204 -0.204 0 0 0 0.238 0.238 0 0 -0.2 0 0 0.374 0 0 0 -0.034 -0.034 0 0 0.275 0.275 0 0 -0.265 -0.265 0 0.096 0 -0.166 -0.166 0 0 0.254 0 0 0 0 0.403 0.403 0 0 0 0 -0.054 0 0 0.172 0 0]
      | sbobj.Groups.Signals(2).Name = 'Signal 2'
      | sbobj.Groups.Signals(2).XData = [0 10]
      | sbobj.Groups.Signals(2).YData = [0 0]
  Signal 1 : Outport  Tag=STV Outport
  Signal 2 : Outport  Tag=STV Outport  Port=2
  wires:
  FromWs/1 -> Demux/1
  Demux/1 -> Signal 1/1
  Demux/2 -> Signal 2/1

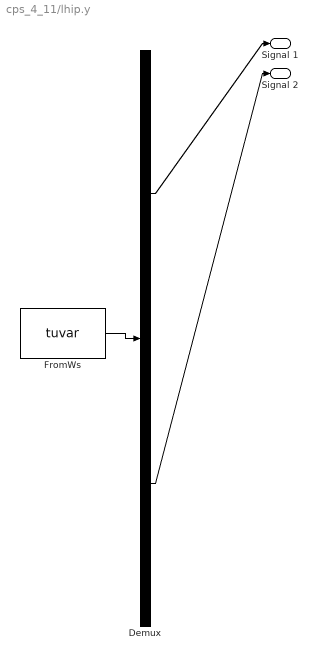
== system cps_4_11/lhip.y ==
  Demux : Demux  Tag=STV Demux  Outputs=2
  FromWs : FromWorkspace  Tag=STV FromWs  VariableName=tuvar  SampleTime=0
      SigBuilderData=|
      | common.afterFinalStr = 'Extrapolate'
      | common.sampleTime = 0
      | dataSet.timeRange = [0 10]
      | dataSet.name = 'Group 1'
      | sbobj.Groups.Name = 'Group 1'
      | sbobj.Groups.Signals(1).Name = 'Signal 1'
      | sbobj.Groups.Signals(1).XData = [0 0.11 0.2 0.33 0.45 0.62 0.62 0.81 0.81 1 1.12 1.29 1.41 1.61 1.76 1.85 1.96 2.05 2.19 2.19 2.33 2.33 2.45 2.45 2.6 2.6 2.73 2.92 3.05 3.24 3.24 3.41 3.41 3.6 3.6 3.81 4 4.1 4.1 4.23 4.23 4.4 4.55 4.55 4.73 4.73 4.89 5.01 5.17 5.39 5.54 5.75 5.89 6 6 6.15 6.15 6.28 6.28 6.45 6.45 6.63 6.63 6.83 6.83 7.05 7.15 7.15 7.31 7.31 7.42 7.59 7.76 7.95 8.13 8.26 8.26 8.42 8.42 8.62 8.78 8.96 9.1 9.31 9.48 9.72 9.89 10]
      | sbobj.Groups.Signals(1).YData = [0 0 0.205 0 0 0 0.1595 0.1595 0 0 0 -0.033 0 0 0.273 0 0 0 0 0.3025 0.3025 0 0 0.32 0.32 0 0 0.197 0 0 0.045 0.045 -0.09 -0.09 0 0 0 0 -0.204 -0.204 0 0 0 0.238 0.238 0 0 -0.2 0 0 0.374 0 0 0 -0.034 -0.034 0 0 0.275 0.275 0 0 -0.265 -0.265 0 0.096 0 -0.166 -0.166 0 0 0.254 0 0 0 0 0.403 0.403 0 0 0 0 -0.054 0 0 0.172 0 0]
      | sbobj.Groups.Signals(2).Name = 'Signal 2'
      | sbobj.Groups.Signals(2).XData = [0 10]
      | sbobj.Groups.Signals(2).YData = [0 0]
  Signal 1 : Outport  Tag=STV Outport
  Signal 2 : Outport  Tag=STV Outport  Port=2
  wires:
  Demux/1 -> Signal 1/1
  FromWs/1 -> Demux/1
  Demux/2 -> Signal 2/1

== system cps_4_11/re.x ==
  Demux : Demux  Tag=STV Demux  Outputs=2
  FromWs : FromWorkspace  Tag=STV FromWs  VariableName=tuvar  SampleTime=0
      SigBuilderData=|
      | common.afterFinalStr = 'Extrapolate'
      | common.sampleTime = 0
      | dataSet.timeRange = [0 10]
      | dataSet.name = 'Group 1'
      | sbobj.Groups.Name = 'Group 1'
      | sbobj.Groups.Signals(1).Name = 'Signal 1'
      | sbobj.Groups.Signals(1).XData = [0 0.11 0.2 0.33 0.45 0.62 0.62 0.81 0.81 1 1.12 1.29 1.41 1.61 1.76 1.85 1.96 2.05 2.19 2.19 2.33 2.33 2.45 2.45 2.6 2.6 2.73 2.92 3.05 3.24 3.24 3.41 3.41 3.6 3.6 3.81 4 4.1 4.1 4.23 4.23 4.4 4.55 4.55 4.73 4.73 4.89 5.01 5.17 5.39 5.54 5.75 5.89 6 6 6.15 6.15 6.28 6.28 6.45 6.45 6.63 6.63 6.83 6.83 7.05 7.15 7.15 7.31 7.31 7.42 7.59 7.76 7.95 8.13 8.26 8.26 8.42 8.42 8.62 8.78 8.96 9.1 9.31 9.48 9.72 9.89 10]
      | sbobj.Groups.Signals(1).YData = [0 0 0.205 0 0 0 0.1595 0.1595 0 0 0 -0.033 0 0 0.273 0 0 0 0 0.3025 0.3025 0 0 0.32 0.32 0 0 0.197 0 0 0.045 0.045 -0.09 -0.09 0 0 0 0 -0.204 -0.204 0 0 0 0.238 0.238 0 0 -0.2 0 0 0.374 0 0 0 -0.034 -0.034 0 0 0.275 0.275 0 0 -0.265 -0.265 0 0.096 0 -0.166 -0.166 0 0 0.254 0 0 0 0 0.403 0.403 0 0 0 0 -0.054 0 0 0.172 0 0]
      | sbobj.Groups.Signals(2).Name = 'Signal 2'
      | sbobj.Groups.Signals(2).XData = [0 10]
      | sbobj.Groups.Signals(2).YData = [0 0]
  Signal 1 : Outport  Tag=STV Outport
  Signal 2 : Outport  Tag=STV Outport  Port=2
  wires:
  Demux/1 -> Signal 1/1
  FromWs/1 -> Demux/1
  Demux/2 -> Signal 2/1

== system cps_4_11/re.y ==
  Demux : Demux  Tag=STV Demux  Outputs=2
  FromWs : FromWorkspace  Tag=STV FromWs  VariableName=tuvar  SampleTime=0
      SigBuilderData=|
      | common.afterFinalStr = 'Extrapolate'
      | common.sampleTime = 0
      | dataSet.timeRange = [0 10]
      | dataSet.name = 'Group 1'
      | sbobj.Groups.Name = 'Group 1'
      | sbobj.Groups.Signals(1).Name = 'Signal 1'
      | sbobj.Groups.Signals(1).XData = [0 0.11 0.2 0.33 0.45 0.62 0.62 0.81 0.81 1 1.12 1.29 1.41 1.61 1.76 1.85 1.96 2.05 2.19 2.19 2.33 2.33 2.45 2.45 2.6 2.6 2.73 2.92 3.05 3.24 3.24 3.41 3.41 3.6 3.6 3.81 4 4.1 4.1 4.23 4.23 4.4 4.55 4.55 4.73 4.73 4.89 5.01 5.17 5.39 5.54 5.75 5.89 6 6 6.15 6.15 6.28 6.28 6.45 6.45 6.63 6.63 6.83 6.83 7.05 7.15 7.15 7.31 7.31 7.42 7.59 7.76 7.95 8.13 8.26 8.26 8.42 8.42 8.62 8.78 8.96 9.1 9.31 9.48 9.72 9.89 10]
      | sbobj.Groups.Signals(1).YData = [0 0 0.205 0 0 0 0.1595 0.1595 0 0 0 -0.033 0 0 0.273 0 0 0 0 0.3025 0.3025 0 0 0.32 0.32 0 0 0.197 0 0 0.045 0.045 -0.09 -0.09 0 0 0 0 -0.204 -0.204 0 0 0 0.238 0.238 0 0 -0.2 0 0 0.374 0 0 0 -0.034 -0.034 0 0 0.275 0.275 0 0 -0.265 -0.265 0 0.096 0 -0.166 -0.166 0 0 0.254 0 0 0 0 0.403 0.403 0 0 0 0 -0.054 0 0 0.172 0 0]
      | sbobj.Groups.Signals(2).Name = 'Signal 2'
      | sbobj.Groups.Signals(2).XData = [0 10]
      | sbobj.Groups.Signals(2).YData = [0 0]
  Signal 1 : Outport  Tag=STV Outport
  Signal 2 : Outport  Tag=STV Outport  Port=2
  wires:
  Demux/1 -> Signal 1/1
  FromWs/1 -> Demux/1
  Demux/2 -> Signal 2/1

== system cps_4_11/rh.x ==
  Demux : Demux  Tag=STV Demux  Outputs=2
  FromWs : FromWorkspace  Tag=STV FromWs  VariableName=tuvar  SampleTime=0
      SigBuilderData=|
      | common.afterFinalStr = 'Extrapolate'
      | common.sampleTime = 0
      | dataSet.timeRange = [0 10]
      | dataSet.name = 'Group 1'
      | sbobj.Groups.Name = 'Group 1'
      | sbobj.Groups.Signals(1).Name = 'Signal 1'
      | sbobj.Groups.Signals(1).XData = [0 0.11 0.2 0.33 0.45 0.62 0.62 0.81 0.81 1 1.12 1.29 1.41 1.61 1.76 1.85 1.96 2.05 2.19 2.19 2.33 2.33 2.45 2.45 2.6 2.6 2.73 2.92 3.05 3.24 3.24 3.41 3.41 3.6 3.6 3.81 4 4.1 4.1 4.23 4.23 4.4 4.55 4.55 4.73 4.73 4.89 5.01 5.17 5.39 5.54 5.75 5.89 6 6 6.15 6.15 6.28 6.28 6.45 6.45 6.63 6.63 6.83 6.83 7.05 7.15 7.15 7.31 7.31 7.42 7.59 7.76 7.95 8.13 8.26 8.26 8.42 8.42 8.62 8.78 8.96 9.1 9.31 9.48 9.72 9.89 10]
      | sbobj.Groups.Signals(1).YData = [0 0 0.205 0 0 0 0.1595 0.1595 0 0 0 -0.033 0 0 0.273 0 0 0 0 0.3025 0.3025 0 0 0.32 0.32 0 0 0.197 0 0 0.045 0.045 -0.09 -0.09 0 0 0 0 -0.204 -0.204 0 0 0 0.238 0.238 0 0 -0.2 0 0 0.374 0 0 0 -0.034 -0.034 0 0 0.275 0.275 0 0 -0.265 -0.265 0 0.096 0 -0.166 -0.166 0 0 0.254 0 0 0 0 0.403 0.403 0 0 0 0 -0.054 0 0 0.172 0 0]
      | sbobj.Groups.Signals(2).Name = 'Signal 2'
      | sbobj.Groups.Signals(2).XData = [0 10]
      | sbobj.Groups.Signals(2).YData = [0 0]
  Signal 1 : Outport  Tag=STV Outport
  Signal 2 : Outport  Tag=STV Outport  Port=2
  wires:
  FromWs/1 -> Demux/1
  Demux/1 -> Signal 1/1
  Demux/2 -> Signal 2/1

== system cps_4_11/rh.y ==
  Demux : Demux  Tag=STV Demux  Outputs=2
  FromWs : FromWorkspace  Tag=STV FromWs  VariableName=tuvar  SampleTime=0
      SigBuilderData=|
      | common.afterFinalStr = 'Extrapolate'
      | common.sampleTime = 0
      | dataSet.timeRange = [0 10]
      | dataSet.name = 'Group 1'
      | sbobj.Groups.Name = 'Group 1'
      | sbobj.Groups.Signals(1).Name = 'Signal 1'
      | sbobj.Groups.Signals(1).XData = [0 0.11 0.2 0.33 0.45 0.62 0.62 0.81 0.81 1 1.12 1.29 1.41 1.61 1.76 1.85 1.96 2.05 2.19 2.19 2.33 2.33 2.45 2.45 2.6 2.6 2.73 2.92 3.05 3.24 3.24 3.41 3.41 3.6 3.6 3.81 4 4.1 4.1 4.23 4.23 4.4 4.55 4.55 4.73 4.73 4.89 5.01 5.17 5.39 5.54 5.75 5.89 6 6 6.15 6.15 6.28 6.28 6.45 6.45 6.63 6.63 6.83 6.83 7.05 7.15 7.15 7.31 7.31 7.42 7.59 7.76 7.95 8.13 8.26 8.26 8.42 8.42 8.62 8.78 8.96 9.1 9.31 9.48 9.72 9.89 10]
      | sbobj.Groups.Signals(1).YData = [0 0 0.205 0 0 0 0.1595 0.1595 0 0 0 -0.033 0 0 0.273 0 0 0 0 0.3025 0.3025 0 0 0.32 0.32 0 0 0.197 0 0 0.045 0.045 -0.09 -0.09 0 0 0 0 -0.204 -0.204 0 0 0 0.238 0.238 0 0 -0.2 0 0 0.374 0 0 0 -0.034 -0.034 0 0 0.275 0.275 0 0 -0.265 -0.265 0 0.096 0 -0.166 -0.166 0 0 0.254 0 0 0 0 0.403 0.403 0 0 0 0 -0.054 0 0 0.172 0 0]
      | sbobj.Groups.Signals(2).Name = 'Signal 2'
      | sbobj.Groups.Signals(2).XData = [0 10]
      | sbobj.Groups.Signals(2).YData = [0.32 0.32]
  Signal 1 : Outport  Tag=STV Outport
  Signal 2 : Outport  Tag=STV Outport  Port=2
  wires:
  Demux/1 -> Signal 1/1
  FromWs/1 -> Demux/1
  Demux/2 -> Signal 2/1

== system cps_4_11/rhip.y ==
  Demux : Demux  Tag=STV Demux  Outputs=2
  FromWs : FromWorkspace  Tag=STV FromWs  VariableName=tuvar  SampleTime=0
      SigBuilderData=|
      | common.afterFinalStr = 'Extrapolate'
      | common.sampleTime = 0
      | dataSet.timeRange = [0 10]
      | dataSet.name = 'Group 1'
      | sbobj.Groups.Name = 'Group 1'
      | sbobj.Groups.Signals(1).Name = 'Signal 1'
      | sbobj.Groups.Signals(1).XData = [0 0.11 0.2 0.33 0.45 0.62 0.62 0.81 0.81 1 1.12 1.29 1.41 1.61 1.76 1.85 1.96 2.05 2.19 2.19 2.33 2.33 2.45 2.45 2.6 2.6 2.73 2.92 3.05 3.24 3.24 3.41 3.41 3.6 3.6 3.81 4 4.1 4.1 4.23 4.23 4.4 4.55 4.55 4.73 4.73 4.89 5.01 5.17 5.39 5.54 5.75 5.89 6 6 6.15 6.15 6.28 6.28 6.45 6.45 6.63 6.63 6.83 6.83 7.05 7.15 7.15 7.31 7.31 7.42 7.59 7.76 7.95 8.13 8.26 8.26 8.42 8.42 8.62 8.78 8.96 9.1 9.31 9.48 9.72 9.89 10]
      | sbobj.Groups.Signals(1).YData = [0 0 0.205 0 0 0 0.1595 0.1595 0 0 0 -0.033 0 0 0.273 0 0 0 0 0.3025 0.3025 0 0 0.32 0.32 0 0 0.197 0 0 0.045 0.045 -0.09 -0.09 0 0 0 0 -0.204 -0.204 0 0 0 0.238 0.238 0 0 -0.2 0 0 0.374 0 0 0 -0.034 -0.034 0 0 0.275 0.275 0 0 -0.265 -0.265 0 0.096 0 -0.166 -0.166 0 0 0.254 0 0 0 0 0.403 0.403 0 0 0 0 -0.054 0 0 0.172 0 0]
      | sbobj.Groups.Signals(2).Name = 'Signal 2'
      | sbobj.Groups.Signals(2).XData = [0 10]
      | sbobj.Groups.Signals(2).YData = [0 0]
  Signal 1 : Outport  Tag=STV Outport
  Signal 2 : Outport  Tag=STV Outport  Port=2
  wires:
  FromWs/1 -> Demux/1
  Demux/1 -> Signal 1/1
  Demux/2 -> Signal 2/1

== system cps_4_11/rs.y ==
  Demux : Demux  Tag=STV Demux  Outputs=2
  FromWs : FromWorkspace  Tag=STV FromWs  VariableName=tuvar  SampleTime=0
      SigBuilderData=|
      | common.afterFinalStr = 'Extrapolate'
      | common.sampleTime = 0
      | dataSet.timeRange = [0 10]
      | dataSet.name = 'Group 1'
      | sbobj.Groups.Name = 'Group 1'
      | sbobj.Groups.Signals(1).Name = 'Signal 1'
      | sbobj.Groups.Signals(1).XData = [0 0.11 0.2 0.33 0.45 0.62 0.62 0.81 0.81 1 1.12 1.29 1.41 1.61 1.76 1.85 1.96 2.05 2.19 2.19 2.33 2.33 2.45 2.45 2.6 2.6 2.73 2.92 3.05 3.24 3.24 3.41 3.41 3.6 3.6 3.81 4 4.1 4.1 4.23 4.23 4.4 4.55 4.55 4.73 4.73 4.89 5.01 5.17 5.39 5.54 5.75 5.89 6 6 6.15 6.15 6.28 6.28 6.45 6.45 6.63 6.63 6.83 6.83 7.05 7.15 7.15 7.31 7.31 7.42 7.59 7.76 7.95 8.13 8.26 8.26 8.42 8.42 8.62 8.78 8.96 9.1 9.31 9.48 9.72 9.89 10]
      | sbobj.Groups.Signals(1).YData = [0 0 0.205 0 0 0 0.1595 0.1595 0 0 0 -0.033 0 0 0.273 0 0 0 0 0.3025 0.3025 0 0 0.32 0.32 0 0 0.197 0 0 0.045 0.045 -0.09 -0.09 0 0 0 0 -0.204 -0.204 0 0 0 0.238 0.238 0 0 -0.2 0 0 0.374 0 0 0 -0.034 -0.034 0 0 0.275 0.275 0 0 -0.265 -0.265 0 0.096 0 -0.166 -0.166 0 0 0.254 0 0 0 0 0.403 0.403 0 0 0 0 -0.054 0 0 0.172 0 0]
      | sbobj.Groups.Signals(2).Name = 'Signal 2'
      | sbobj.Groups.Signals(2).XData = [0 10]
      | sbobj.Groups.Signals(2).YData = [0 0]
  Signal 1 : Outport  Tag=STV Outport
  Signal 2 : Outport  Tag=STV Outport  Port=2
  wires:
  FromWs/1 -> Demux/1
  Demux/1 -> Signal 1/1
  Demux/2 -> Signal 2/1

== matlab function cps_4_11/Stop System/value of stop ==
  data: y output; stop data_store_memory
function y = fcn
%#codegen
global stop;
y=stop;

== matlab function cps_4_11/Stop System/stop++ ==
  data: u input; stop data_store_memory
function fcn(u)
%#codegen
global stop;
stop=stop+u;

== matlab function cps_4_11/Forward System/value of forwarda ==
  data: y output; forwarda data_store_memory
function y = fcn
%#codegen
global forwarda;
y = forwarda;

== matlab function cps_4_11/Forward System/reset backwarda and backwardb ==
  data: u input; backwarda data_store_memory; backwardb data_store_memory
function fcn(u)
%#codegen
global backwarda;
global backwardb;
if (u==1)
    backwarda=0;
    backwardb=0;
end

== matlab function cps_4_11/Forward System/set forwardb=1 ==
  data: u input; forwardb data_store_memory
function fcn(u)
%#codegen
global forwardb;
if u==1
    forwardb=1;
end

== matlab function cps_4_11/Stop System/reset backwarda and backwardb ==
  data: u input; backwarda data_store_memory; backwardb data_store_memory
function fcn(u)
%#codegen
global backwarda;
global backwardb;
if (u==1)
    backwarda=0;
    backwardb=0;
end

== matlab function cps_4_11/Forward System/value of forwardb ==
  data: y output; forwardb data_store_memory
function y = fcn
%#codegen
global forwardb;
y = forwardb;

== matlab function cps_4_11/Forward System/set forwarda=2 ==
  data: u input; forwarda data_store_memory
function fcn(u)
%#codegen
global forwarda;
if u==1
    forwarda=2;
end

== matlab function cps_4_11/Forward System/set forwarda=1 ==
  data: u input; forwarda data_store_memory
function fcn(u)
%#codegen
global forwarda;
if u==1
    forwarda=1;
end

== matlab function cps_4_11/Backward System/value of backwarda ==
  data: y output; backwarda data_store_memory
function y = fcn
%#codegen
global backwarda;
y = backwarda;

== matlab function cps_4_11/Backward System/set forwarda, forwardb, autoa, and autob to 0 ==
  data: u input; forwarda data_store_memory; forwardb data_store_memory; autoa data_store_memory; autob data_store_memory
function fcn(u)
%#codegen
global forwarda;
global forwardb;
global autoa;
global autob;
if u==1
    forwarda=0;
    forwardb=0;
    autoa=0;
    autob=0;
end

== matlab function cps_4_11/Backward System/set backwardb=1 ==
  data: u input; backwardb data_store_memory
function fcn(u)
%#codegen
global backwardb;
if u==1
    backwardb=1;
end

== matlab function cps_4_11/Backward System/value of backwardb ==
  data: y output; backwardb data_store_memory
function y = fcn
%#codegen
global backwardb;
y=backwardb;

== matlab function cps_4_11/Backward System/set backwarda=2 ==
  data: u input; backwarda data_store_memory
function fcn(u)
%#codegen
global backwarda;
if u==1
    backwarda=2;
end

== matlab function cps_4_11/Backward System/set backwarda=1 ==
  data: u input; backwarda data_store_memory
function fcn(u)
%#codegen
global backwarda;
if u==1
    backwarda=1;
end

== matlab function cps_4_11/Auto System/value of autoa ==
  data: y output; autoa data_store_memory
function y = fcn
%#codegen
global autoa;
y=autoa;

== matlab function cps_4_11/Auto System/set autob=1 ==
  data: u input; autob data_store_memory
function fcn(u)
%#codegen
global autob;
if u==1
    autob=1;
end

== matlab function cps_4_11/Auto System/set mana and manb to 0 ==
  data: u input; mana data_store_memory; manb data_store_memory
function fcn(u)
%#codegen
global mana;
global manb;
if u==1
    mana=0;
    manb=0;
end

== matlab function cps_4_11/Auto System/value of autob ==
  data: y output; autob data_store_memory
function y = fcn
%#codegen
global autob;
y = autob;

== matlab function cps_4_11/Auto System/set autoa to 2 ==
  data: u input; autoa data_store_memory
function fcn(u)
%#codegen
global autoa;
if u==1
    autoa=2;
end

== matlab function cps_4_11/Auto System/set autoa to 1 ==
  data: u input; autoa data_store_memory
function fcn(u)
%#codegen
global autoa
if u==1
    autoa=1;
end

== matlab function cps_4_11/Manual System/set mana to 1 ==
  data: u input; mana data_store_memory
function fcn(u)
%#codegen
global mana
if u==1
    mana=1;
end

== matlab function cps_4_11/Manual System/set mana to 2 ==
  data: u input; mana data_store_memory
function fcn(u)
%#codegen
global mana;
if u==1
    mana=2;
end

== matlab function cps_4_11/Manual System/set manb=1 ==
  data: u input; manb data_store_memory
function fcn(u)
%#codegen
global manb;
if u==1
    manb=1;
end

== matlab function cps_4_11/Manual System/set autoa and autob to 0 ==
  data: u input; autoa data_store_memory; autob data_store_memory
function fcn(u)
%#codegen
global autoa;
global autob;
if u==1
    autoa=0;
    autob=0;
end

== matlab function cps_4_11/Manual System/value of mana ==
  data: y output; mana data_store_memory
function y = fcn
%#codegen
global mana;
y=mana;

== matlab function cps_4_11/Manual System/value of manb ==
  data: y output; manb data_store_memory
function y = fcn
%#codegen
global manb;
y = manb;

== matlab function cps_4_11/Turning System/increment turncount set all others to 0 ==
  data: u input; backwarda data_store_memory; backwardb data_store_memory; forwarda data_store_memory; forwardb data_store_memory; autoa data_store_memory; autob data_store_memory; mana data_store_memory; manb data_store_memory; stop data_store_memory; turncount data_store_memory
function fcn(u)
%#codegen
global backwarda;
global backwardb;
global forwarda;
global forwardb;
global autoa;
global autob;
global mana;
global manb;
global stop;
global turncount;
if u==1
    backwarda=0;
    backwardb=0;
    forwarda=0;
    forwardb=0;
    autoa=0;
    autob=0;
    mana=0;
    manb=0;
    stop=0;
    turncount=turncount+1;
end

== matlab function cps_4_11/Turning System/first add current result to total, then if turncount==10,  ==
  data: u input; y output; turncount data_store_memory; result data_store_memory
function y = fcn(u)
%#codegen
global result;
global turncount;
result=result+u;
y=0;
if turncount==10
    y=result/10;
end

== matlab function cps_4_11/if so, clear all variables ==
  data: u input; stop data_store_memory; forwarda data_store_memory; forwardb data_store_memory; backwarda data_store_memory; backwardb data_store_memory; autoa data_store_memory; autob data_store_memory; mana data_store_memory; manb data_store_memory; result data_store_memory; turncount data_store_memory
function fcn(u)
%#codegen
global stop;
global forwarda;
global forwardb;
global backwarda;
global backwardb;
global autoa;
global autob;
global mana;
global manb;
global result;
global turncount;
if u==1
    stop = 0;
	forwarda = 0;
	forwardb = 0;
	backwarda = 0;
	backwardb = 0;
	autoa = 0;
	autob = 0;
	mana = 0;
	manb = 0;
	result = 0;
	turncount = 0;
end

== matlab function cps_4_11/When sensor triggers, pause for x seconds ==
  data: u input; y output
function y = fcn(u)
%#codegen
y=false;
if u==true
    pause(0.1);
    y=true;
end

== stateflow chart cps_4_11/Robot Model ==
  state Manual
    state Avoid_Obstacle
      en: backup=1;
      ex: backup=0;
    state Stop
      state Stop
      state TurnL
      state TurnR
      (default) -> Manual.Stop.Stop
      Manual.Stop.Stop -> Manual.Stop.TurnR [order 2] : [result<0]
      Manual.Stop.Stop -> Manual.Stop.TurnL [order 1] : [result>0]
      Manual.Stop.TurnL -> Manual.Stop.Stop [order 1] : [result==0]
      Manual.Stop.TurnR -> Manual.Stop.Stop [order 1] : [result==0]
      Manual.Stop.TurnL -> Manual.Stop.TurnR [order 2] : [result<0]
      Manual.Stop.TurnR -> Manual.Stop.TurnL [order 2] : [result>0]
    state Backward
      state Backward
      state TurnL
      state TurnR
      (default) -> Manual.Backward.Backward
      Manual.Backward.Backward -> Manual.Backward.TurnR [order 2] : [result<0]
      Manual.Backward.Backward -> Manual.Backward.TurnL [order 1] : [result>0]
      Manual.Backward.TurnL -> Manual.Backward.Backward [order 1] : [result==0]
      Manual.Backward.TurnR -> Manual.Backward.Backward [order 1] : [result==0]
      Manual.Backward.TurnL -> Manual.Backward.TurnR [order 2] : [result<0]
      Manual.Backward.TurnR -> Manual.Backward.TurnL [order 2] : [result>0]
    state Forward
      state Forward
      state TurnL
      state TurnR
      (default) -> Manual.Forward.Forward
      Manual.Forward.Forward -> Manual.Forward.TurnR [order 2] : [result<0]
      Manual.Forward.Forward -> Manual.Forward.TurnL [order 1] : [result>0]
      Manual.Forward.TurnL -> Manual.Forward.Forward [order 1] : [result==0]
      Manual.Forward.TurnR -> Manual.Forward.Forward [order 1] : [result==0]
      Manual.Forward.TurnL -> Manual.Forward.TurnR [order 2] : [result<0]
      Manual.Forward.TurnR -> Manual.Forward.TurnL [order 2] : [result>0]
    Manual.Backward -> Avoid_Obstacle [order 1] : [wall==1 || left_sensor==1 || right_sensor==1]
    Manual.Stop -> Avoid_Obstacle [order 1] : [wall==1 || left_sensor==1 || right_sensor==1]
    (default) -> Avoid_Obstacle [order 1] : [wall==1 || left_sensor==1 || right_sensor==1]
    Avoid_Obstacle -> Manual.Stop : [wall==0 && left_sensor==0 && right_sensor==0 && delay_done]
    (default) -> Manual.Stop [order 2]
    Manual.Stop -> Manual.Forward [order 3] : [goforward==1]
    Manual.Backward -> Manual.Stop [order 2] : [stop==1]
    Manual.Forward -> Manual.Stop [order 1] : [stop==1]
    Manual.Stop -> Manual.Backward [order 2] : [backward==1]
    Manual.Backward -> Manual.Forward [order 3] : [goforward==1]
    Manual.Forward -> Manual.Backward [order 2] : [backward==1]
  state Auto
    state Forward
    state Backward
      en:backup=1;
    state TurnL
      en:backup=0;
      turnl=1;
      ex:turnl=0;
    state TurnR
      en:backup=0;
      turnr=1;
      ex:turnr=0;
    Auto.TurnL -> Auto.Forward [order 1] : [right_sensor==0 && wall==0 && left_sensor==0 && delay_done1]
    (default) -> Auto.Forward
    Auto.TurnR -> Auto.Forward [order 1] : [right_sensor==0 && wall==0 && left_sensor==0 && delay_done1]
    Auto.Forward -> Auto.Backward : [right_sensor==1 || wall==1 || left_sensor==1]
    Auto.Backward -> Auto.TurnR [order 2] : [delay_done]
    Auto.Backward -> Auto.TurnL [order 1] : [delay_done]
    Auto.TurnR -> Auto.Backward [order 2] : [delay_done1 && (right_sensor==1 || wall==1 || left_sensor==1)]
    Auto.TurnL -> Auto.Backward [order 2] : [delay_done1 && (right_sensor==1 || wall==1 || left_sensor==1)]
  (default) -> Manual
  Auto -> Manual : [manual==1]
  Manual -> Auto : [auto==1]
  data: goforward input; backward input; stop input; manual input; auto input; result input; wall input double size=1; right_sensor input double size=1; left_sensor input double size=1; delay_done input boolean size=1; delay_done1 input boolean size=1; backup output double size=1; turnr output double size=1; turnl output double size=1

== matlab function cps_4_11/When sensor triggers, pause for x seconds2 ==
  data: u input; y output
function y = fcn(u)
%#codegen
y=false;
if u==true
    pause(0.1);
    y=true;
end

== matlab function cps_4_11/When sensor triggers, pause for x seconds1 ==
  data: u input; y output
function y = fcn(u)
%#codegen
y=false;
if u==true
    pause(0.1);
    y=true;
end
